simulink model "lowpass"  (R2013a)
settings: Solver=ode45  StartTime=0.0  StopTime=599.0  RelTol=1e-3
undefined symbols (not defined in the file or in its folder): dfilt, fdesignblkfcn, gcbh
libraries: dsparch4 x3
settings Model: Creator=不会起名字  LastModifiedBy=不会起名字

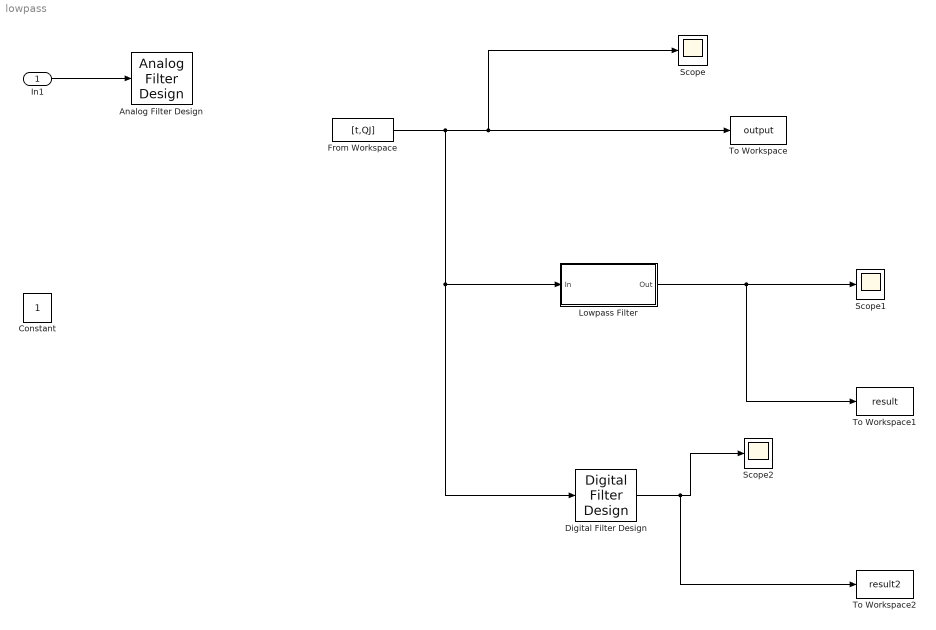
== system lowpass ==
  In1 : Inport
  Analog Filter Design : dsparch4/Analog Filter Design  method=Butterworth  filttype=Lowpass  N=8  Wlo=30  Whi=80  Rp=2  Rs=40
  Constant : Constant
  Digital Filter Design : dsparch4/Digital Filter Design  mwdsp_browser_bugfix_var=off
  From Workspace : FromWorkspace  VariableName=[t,QJ]  SampleTime=1  OutputAfterFinalValue=Holding final value
  Lowpass Filter : Subsystem  DialogController=fdesignblkfcn  InitFcn=fdesignblkfcn(gcbh, {'InitFcn'});  mask(Lowpass Filter){}
      mask help: Design a lowpass filter
      settings: CopyFcn=fdesignblkfcn(gcbh, {'CopyFcn'});
      mask Help: helpview(mapfilelocation('dsp'), 'dsplowpassfilter');
      mask Display: disp('Lowpass')
  Scope : Scope
      settings: TimeRange=600  YMin=-500  YMax=1500
  Scope1 : Scope
  Scope2 : Scope
      settings: SaveName=ScopeData2
  To Workspace : ToWorkspace  VariableName=output  SampleTime=-1  SaveFormat=Timeseries
  To Workspace1 : ToWorkspace  VariableName=result  SampleTime=-1  SaveFormat=Timeseries
  To Workspace2 : ToWorkspace  VariableName=result2  SampleTime=-1  SaveFormat=Timeseries
  wires:
  From Workspace/1 -> Digital Filter Design/1, Lowpass Filter/1(In), To Workspace/1, Scope/1
  Lowpass Filter/1(Out) -> To Workspace1/1, Scope1/1
  Digital Filter Design/1 -> To Workspace2/1, Scope2/1
  In1/1 -> Analog Filter Design/1

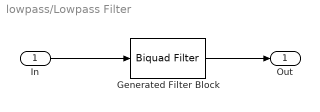
== system lowpass/Lowpass Filter ==
  In : Inport
  Generated Filter Block : dsparch4/Biquad Filter  Tag=BlockMethodSubSystem  IIRFiltStruct=Direct form II  CoeffSource=Specify via dialog  BiQuadCoeffs=[0.35230146550854152 0.70460293101708305 0.35230146550854152 1 -0.18062861276293468 0.53038926211178405;0.37244578900933756 0.74489157801867512 0.37244578900933756 1 -0.13693336440674406 0.16017804326471285;0.29855268988135275 0.5971053797627055 0.29855268988135275 1 -0.12032531746022769 0.019465138909104326;0.47159705718998224 0.47159705718998224 0 1 -0.059220912888930811 0;0.28757913514155453 0.57515827028310906 0.28757913514155453 1 -0.12622078183180585 0.069414896211770119;0.12715010224927567 0.25430020449855134 0.12715010224927567 1 -0.15407520680966669 0.30541356904863526;0.25769180793642382 0.51538361587284764 0.25769180793642382 1 -0.22220117092993169 0.88261583155784673;0.38371715199711864 0.76743430399423729 0.38371715199711864 1 -0.16590894239324383 0.40567576777096676;0.4241945043675025 0.848389008735005 0.4241945043675025 1 -0.13089759638917958 0.10903955295918411;0.30073110142976406 0.60146220285952812 0.30073110142976406 1 -0.11890899806690422 0.007465268245713438;0.2700517711378963 0.5401035422757926 0.2700517711378963 1 -0.12273619539171698 0.039891480241060456;0.22383459775733791 0.44766919551467582 0.22383459775733791 1 -0.14455622726397821 0.2247633118155635;0.41526636234151509 0.83053272468303019 0.41526636234151509 1 -0.1990232141590243 0.6862388809888802]  a0Flag=Warning  IC=0  ICnum=0  ICden=0  InputProcessing=Columns as channels (frame based)  denAccumFracLength=30  denProdOutputFracLength=30  secondMemoryFracLength=15  roundingMode=Floor  overflowMode=off  ScaleValues=[0.46598578007750174;1;1;1;1;1;1;1;1;1;1;1;1;1]  optimizeScaleValues=off  ScaleValueMode=Specify via input port (g)  scaleValueFracLength=14  FilterSource=Specify via dialog  dfiltObjectName=dfilt.df2tsos([1 0.3 0.4],[1 0.1 0.2])
  Out : Outport
  wires:
  In/1 -> Generated Filter Block/1
  Generated Filter Block/1 -> Out/1
